simulink model "Ohms_Law"  (R2024b)
settings: Solver=VariableStepAuto  StartTime=0.0  StopTime=10.0  RelTol=1e-3
libraries: spsVoltageMeasurementLib x20, spsSeriesRLCBranchLib x14, spsCurrentMeasurementLib x6, spsACVoltageSourceLib x5, spsDCVoltageSourceLib x1, spspowerguiLib x1
settings Model: Creator=priya  LastModifiedBy=priya

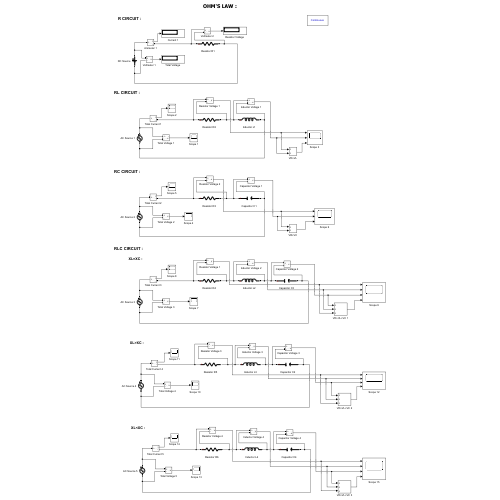
[thumbnail: Simulink's stored preview of the top-level diagram]
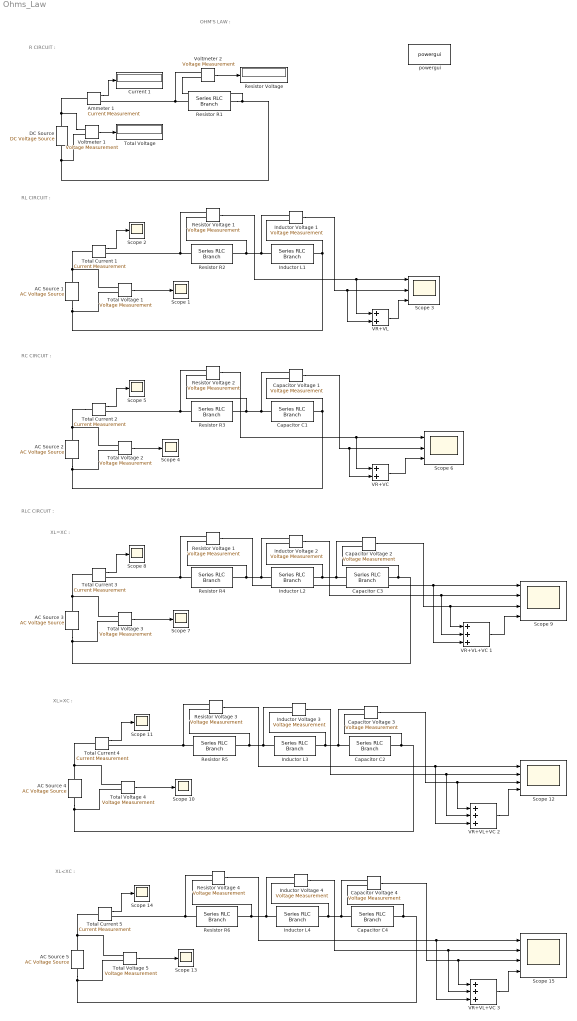
== system Ohms_Law ==
  note: OHM'S LAW :
  note: R CIRCUIT :
  note: RL CIRCUIT :
  note: RC CIRCUIT :
  note: RLC CIRCUIT :
  note: XL=XC :
  note: XL>XC :
  note: XL<XC :
  AC Source {1..5} (5 alike) : spsACVoltageSourceLib/AC Voltage Source  Amplitude=50  Phase=0  Frequency=60  SampleTime=0  Measurements=None  BusType=swing  Pref=10e3  Qref=0  Qmin=-inf  Qmax=+inf
  Ammeter 1 : spsCurrentMeasurementLib/Current Measurement  PhasorSimulation=off  OutputType=Complex  PSBequivalent=0
  Capacitor C1 : spsSeriesRLCBranchLib/Series RLC Branch  LConnTagsString=__new0  RConnTagsString=__new0  BranchType=C  Resistance=1  Inductance=1  SetiL0=off  InitialCurrent=0  Capacitance=0.0015  Setx0=off  InitialVoltage=0  Measurements=None
  Capacitor C2 : spsSeriesRLCBranchLib/Series RLC Branch  LConnTagsString=__new0  RConnTagsString=__new0  BranchType=C  Resistance=1  Inductance=1  SetiL0=off  InitialCurrent=0  Capacitance=0.0015  Setx0=off  InitialVoltage=0  Measurements=None
  Capacitor C3 : spsSeriesRLCBranchLib/Series RLC Branch  LConnTagsString=__new0  RConnTagsString=__new0  BranchType=C  Resistance=1  Inductance=1  SetiL0=off  InitialCurrent=0  Capacitance=7.04e-4  Setx0=off  InitialVoltage=0  Measurements=None
  Capacitor C4 : spsSeriesRLCBranchLib/Series RLC Branch  LConnTagsString=__new0  RConnTagsString=__new0  BranchType=C  Resistance=1  Inductance=1  SetiL0=off  InitialCurrent=0  Capacitance=100e-6  Setx0=off  InitialVoltage=0  Measurements=None
  Capacitor Voltage {1..4} (4 alike) : spsVoltageMeasurementLib/Voltage Measurement  PhasorSimulation=off  OutputType=Complex  PSBequivalent=0
  Current 1 : Display
  DC Source : spsDCVoltageSourceLib/DC Voltage Source  Amplitude=50  Measurements=None
  Inductor L1 : spsSeriesRLCBranchLib/Series RLC Branch  LConnTagsString=__new0  RConnTagsString=__new0  BranchType=L  Resistance=1  Inductance=0.01  SetiL0=off  InitialCurrent=0  Capacitance=1e-6  Setx0=off  InitialVoltage=0  Measurements=None
  Inductor L2 : spsSeriesRLCBranchLib/Series RLC Branch  LConnTagsString=__new0  RConnTagsString=__new0  BranchType=L  Resistance=1  Inductance=0.01  SetiL0=off  InitialCurrent=0  Capacitance=100e-6  Setx0=off  InitialVoltage=0  Measurements=None
  Inductor L3 : spsSeriesRLCBranchLib/Series RLC Branch  LConnTagsString=__new0  RConnTagsString=__new0  BranchType=L  Resistance=1  Inductance=0.01  SetiL0=off  InitialCurrent=0  Capacitance=100e-6  Setx0=off  InitialVoltage=0  Measurements=None
  Inductor L4 : spsSeriesRLCBranchLib/Series RLC Branch  LConnTagsString=__new0  RConnTagsString=__new0  BranchType=L  Resistance=1  Inductance=0.01  SetiL0=off  InitialCurrent=0  Capacitance=100e-6  Setx0=off  InitialVoltage=0  Measurements=None
  Inductor Voltage {1..4} (4 alike) : spsVoltageMeasurementLib/Voltage Measurement  PhasorSimulation=off  OutputType=Complex  PSBequivalent=0
  Resistor R1 : spsSeriesRLCBranchLib/Series RLC Branch  LConnTagsString=__new0  RConnTagsString=__new0  BranchType=R  Resistance=20  Inductance=1e-3  SetiL0=off  InitialCurrent=0  Capacitance=1e-6  Setx0=off  InitialVoltage=0  Measurements=None
  Resistor R{2..6} (5 alike) : spsSeriesRLCBranchLib/Series RLC Branch  LConnTagsString=__new0  RConnTagsString=__new0  BranchType=R  Resistance=10  Inductance=1e-3  SetiL0=off  InitialCurrent=0  Capacitance=1e-6  Setx0=off  InitialVoltage=0  Measurements=None
  "Resistor Voltage " : Display
  Resistor Voltage {1..4} (4 alike) : spsVoltageMeasurementLib/Voltage Measurement  PhasorSimulation=off  OutputType=Complex  PSBequivalent=0
  "Resistor Voltage 1 " : spsVoltageMeasurementLib/Voltage Measurement  PhasorSimulation=off  OutputType=Complex  PSBequivalent=0
  Scope {1..2,4..5,7..8,10..11,13..14} (10 alike) : Scope
  Scope 12 : Scope  NumInputPorts=4
  Scope 15 : Scope  NumInputPorts=4
  "Scope 3 " : Scope  NumInputPorts=3
  Scope 6 : Scope  NumInputPorts=3
  Scope 9 : Scope  NumInputPorts=4
  Total Current {1..4} (4 alike) : spsCurrentMeasurementLib/Current Measurement  PhasorSimulation=off  OutputType=Complex  PSBequivalent=0
  "Total Current 5 " : spsCurrentMeasurementLib/Current Measurement  PhasorSimulation=off  OutputType=Complex  PSBequivalent=0
  "Total Voltage " : Display
  Total Voltage {1..5} (5 alike) : spsVoltageMeasurementLib/Voltage Measurement  PhasorSimulation=off  OutputType=Complex  PSBequivalent=0
  VR+VC : Sum
  VR+VL : Sum
  VR+VL+VC 1 : Sum  Inputs=+++
  VR+VL+VC 2 : Sum  Inputs=+++
  VR+VL+VC 3 : Sum  Inputs=+++
  Voltmeter 1 : spsVoltageMeasurementLib/Voltage Measurement  PhasorSimulation=off  OutputType=Complex  PSBequivalent=0
  Voltmeter 2 : spsVoltageMeasurementLib/Voltage Measurement  PhasorSimulation=off  OutputType=Complex  PSBequivalent=0
  powergui : spspowerguiLib/powergui  Priority=1  SimulationMode=Continuous  SampleTime=50e-6  frequency=60  Iterations=50  frequencyindice=0  Pbase=100e6  ErrMax=1e-4  UnitsV=kV  UnitsW=MW  buscounter=0  FunctionMessages=off  echomessages=off  EnableUseOfTLC=off  CurrentSourceSwitches=off  DisableSnubberDevices=off  DisableRonSwitches=off  DisableVfSwitches=off  DisplayEquations=off  AutomaticDiscreteSolvers=off  SolverType=Tustin/Backward Euler (TBE)  Interpol=off  ExternalGateDelay=off  methode=off  Ts=100  x0status=blocks  SPID=on  SwTol=0  HookPort=off  NonlinearTolerance=1e-4  nMaxIteration=100  ContinueOnMaxIteration=off  RestoreLinks=warning  ResistiveCurrentMeasurement=off  Frange=[0:2:500]  Ylog=off  Xlog=on  ShowGrid=off  save=off  variable=ZData  structure=0  ZoomFFT=off  StartTime=0.0  cycles=1  DisplayStyle=1  fundamental=60  FreqAxis=off  MaxFrequency=1000  frequencyindicesteady=1  RmsSteady=1  display=off
  wires:
  Voltmeter 1/1 -> "Total Voltage "/1
  Ammeter 1/1 -> Current 1/1
  Voltmeter 2/1 -> "Resistor Voltage "/1
  Total Current 1/1 -> Scope 2/1
  Total Voltage 1/1 -> Scope 1/1
  "Resistor Voltage 1 "/1 -> VR+VL/1, "Scope 3 "/1
  Inductor Voltage 1/1 -> VR+VL/2, "Scope 3 "/2
  Capacitor Voltage 1/1 -> VR+VC/2, Scope 6/2
  Resistor Voltage 2/1 -> VR+VC/1, Scope 6/1
  Total Voltage 2/1 -> Scope 4/1
  Total Current 2/1 -> Scope 5/1
  Total Current 3/1 -> Scope 8/1
  Total Voltage 3/1 -> Scope 7/1
  Capacitor Voltage 2/1 -> VR+VL+VC 1/1, Scope 9/3
  Inductor Voltage 2/1 -> VR+VL+VC 1/2, Scope 9/2
  Resistor Voltage 1/1 -> VR+VL+VC 1/3, Scope 9/1
  Total Current 4/1 -> Scope 11/1
  Resistor Voltage 3/1 -> VR+VL+VC 2/3, Scope 12/1
  Capacitor Voltage 3/1 -> VR+VL+VC 2/1, Scope 12/3
  Total Voltage 4/1 -> Scope 10/1
  Inductor Voltage 4/1 -> VR+VL+VC 3/2, Scope 15/2
  "Total Current 5 "/1 -> Scope 14/1
  Resistor Voltage 4/1 -> VR+VL+VC 3/3, Scope 15/1
  Capacitor Voltage 4/1 -> VR+VL+VC 3/1, Scope 15/3
  Total Voltage 5/1 -> Scope 13/1
  VR+VL/1 -> "Scope 3 "/3
  VR+VC/1 -> Scope 6/3
  VR+VL+VC 1/1 -> Scope 9/4
  Inductor Voltage 3/1 -> VR+VL+VC 2/2, Scope 12/2
  VR+VL+VC 2/1 -> Scope 12/4
  VR+VL+VC 3/1 -> Scope 15/4
  connections:
  Voltmeter 1/LConn1 -- DC Source/RConn1 -- Ammeter 1/LConn1
  AC Source 1/RConn1 -- Total Voltage 1/LConn1 -- Total Current 1/LConn1
  Resistor R2/LConn1 -- "Resistor Voltage 1 "/LConn1 -- Total Current 1/RConn1
  Inductor L1/LConn1 -- "Resistor Voltage 1 "/LConn2 -- Resistor R2/RConn1 -- Inductor Voltage 1/LConn1
  Resistor R1/LConn1 -- Voltmeter 2/LConn1 -- Ammeter 1/RConn1
  Resistor R1/RConn1 -- Voltmeter 2/LConn2 -- Voltmeter 1/LConn2 -- DC Source/LConn1
  AC Source 1/LConn1 -- Total Voltage 1/LConn2 -- Inductor Voltage 1/LConn2 -- Inductor L1/RConn1
  Resistor R3/LConn1 -- Resistor Voltage 2/LConn1 -- Total Current 2/RConn1
  Capacitor C1/RConn1 -- Total Voltage 2/LConn2 -- AC Source 2/LConn1 -- Capacitor Voltage 1/LConn2
  Resistor R3/RConn1 -- Capacitor Voltage 1/LConn1 -- Capacitor C1/LConn1 -- Resistor Voltage 2/LConn2
  Total Current 2/LConn1 -- AC Source 2/RConn1 -- Total Voltage 2/LConn1
  Resistor R4/RConn1 -- Resistor Voltage 1/LConn2 -- Inductor Voltage 2/LConn1 -- Inductor L2/LConn1
  Total Voltage 3/LConn1 -- Total Current 3/LConn1 -- AC Source 3/RConn1
  Inductor Voltage 2/LConn2 -- Capacitor Voltage 2/LConn1 -- Capacitor C3/LConn1 -- Inductor L2/RConn1
  Resistor R4/LConn1 -- Resistor Voltage 1/LConn1 -- Total Current 3/RConn1
  AC Source 3/LConn1 -- Total Voltage 3/LConn2 -- Capacitor Voltage 2/LConn2 -- Capacitor C3/RConn1
  AC Source 4/RConn1 -- Total Voltage 4/LConn1 -- Total Current 4/LConn1
  Inductor L3/LConn1 -- Resistor R5/RConn1 -- Resistor Voltage 3/LConn2 -- Inductor Voltage 3/LConn1
  Capacitor C2/RConn1 -- AC Source 4/LConn1 -- Total Voltage 4/LConn2 -- Capacitor Voltage 3/LConn2
  Total Current 4/RConn1 -- Resistor R5/LConn1 -- Resistor Voltage 3/LConn1
  Capacitor C2/LConn1 -- Inductor Voltage 3/LConn2 -- Inductor L3/RConn1 -- Capacitor Voltage 3/LConn1
  AC Source 5/RConn1 -- Total Voltage 5/LConn1 -- "Total Current 5 "/LConn1
  Inductor L4/LConn1 -- Resistor R6/RConn1 -- Resistor Voltage 4/LConn2 -- Inductor Voltage 4/LConn1
  Capacitor C4/RConn1 -- AC Source 5/LConn1 -- Total Voltage 5/LConn2 -- Capacitor Voltage 4/LConn2
  "Total Current 5 "/RConn1 -- Resistor R6/LConn1 -- Resistor Voltage 4/LConn1
  Capacitor C4/LConn1 -- Inductor Voltage 4/LConn2 -- Inductor L4/RConn1 -- Capacitor Voltage 4/LConn1
